simulink model "segway_TP3_sensors"  (R2016a)
settings: Solver=VariableStepAuto  StartTime=t0  StopTime=200  FixedStep=h  RelTol=1e-3
values from neighbouring files (symbols this model uses):
  h = (tf-t0)/N    [init.m]    (also in init_tp3.m)
  l = 10    [init.m]    (also in init_TP1.m = 1; init_TP2_controle.m; init_tp3.m = 5)
undefined symbols (not defined in the file or in its folder): DiscIntNeverNeededParam
libraries: simulink x1
settings Model: Creator=fgaribal  LastModifiedBy=fgaribal

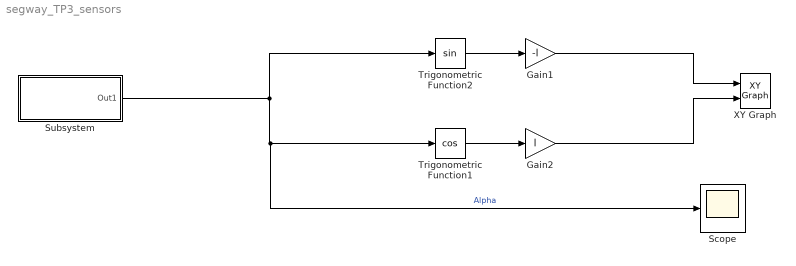
== system segway_TP3_sensors ==
  Gain1 : Gain  Gain=-l
  Gain2 : Gain  Gain=l
  Scope : Scope
  Subsystem : Subsystem
  Trigonometric Function1 : Trigonometry  Operator=cos
  Trigonometric Function2 : Trigonometry
  XY Graph : simulink/Sinks/XY Graph  xmin=-l  xmax=l  ymin=-l  ymax=l  st=-1
  wires:
  Trigonometric Function1/1 -> Gain2/1
  Trigonometric Function2/1 -> Gain1/1
  Gain2/1 -> XY Graph/2
  Gain1/1 -> XY Graph/1
  Subsystem/1(Out1) -> Scope/1, Trigonometric Function1/1, Trigonometric Function2/1  "Alpha"

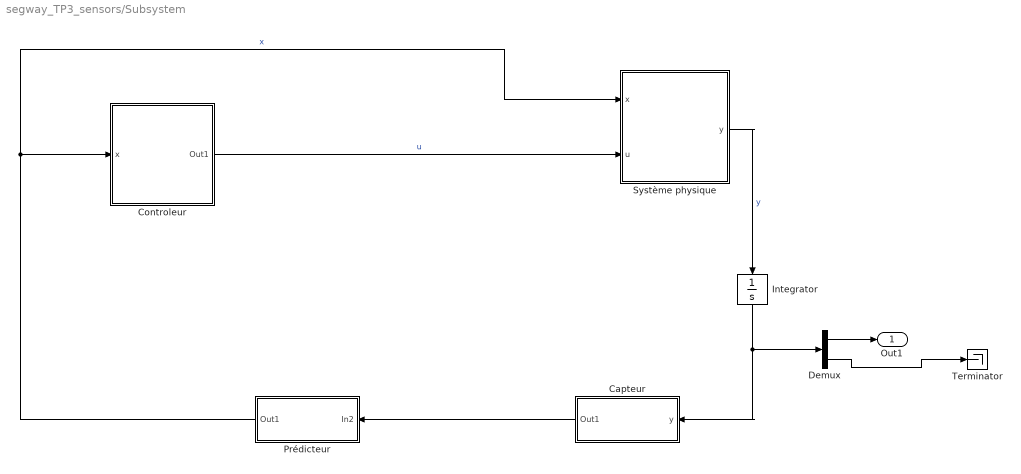
== system segway_TP3_sensors/Subsystem ==
  "Capteur " : Subsystem
  Controleur : Subsystem
  Demux : Demux  Outputs=2
  Integrator : Integrator  InitialCondition=pi/4
  Prédicteur : Subsystem
  Système physique : Subsystem
  Terminator : Terminator
  Out1 : Outport
  wires:
  Controleur/1(Out1) -> Système physique/2(u)  "u"
  Prédicteur/1(Out1) -> Système physique/1(x), Controleur/1(x)  "x"
  Système physique/1(y) -> Integrator/1  "y"
  "Capteur "/1(Out1) -> Prédicteur/1(In2)
  Integrator/1 -> Demux/1, "Capteur "/1(y)
  Demux/1 -> Out1/1
  Demux/2 -> Terminator/1

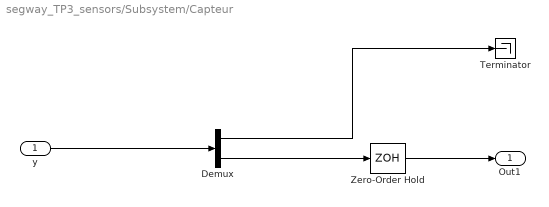
== system segway_TP3_sensors/Subsystem/Capteur  ==
  y : Inport
  Demux : Demux  Outputs=2
  Terminator : Terminator
  Zero-Order Hold : ZeroOrderHold  SampleTime=25*h
  Out1 : Outport
  wires:
  Demux/2 -> Zero-Order Hold/1
  Demux/1 -> Terminator/1
  y/1 -> Demux/1
  Zero-Order Hold/1 -> Out1/1

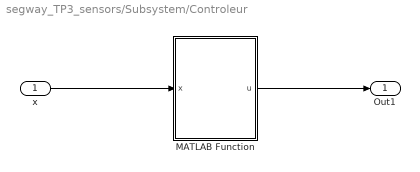
== system segway_TP3_sensors/Subsystem/Controleur ==
  x : Inport
  MATLAB Function : MATLAB Function  TreatAsAtomicUnit=on
  Out1 : Outport
  wires:
  MATLAB Function/1(u) -> Out1/1
  x/1 -> MATLAB Function/1(x)

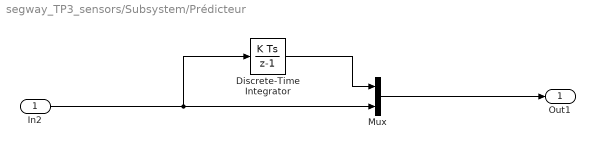
== system segway_TP3_sensors/Subsystem/Prédicteur ==
  In2 : Inport
  Discrete-Time Integrator : DiscreteIntegrator  InitialConditionSetting=State (most efficient)  SampleTime=25*h  ICPrevOutput=DiscIntNeverNeededParam  ICPrevScaledInput=DiscIntNeverNeededParam
  Mux : Mux  Inputs=2
  Out1 : Outport
  wires:
  In2/1 -> Discrete-Time Integrator/1, Mux/2
  Discrete-Time Integrator/1 -> Mux/1
  Mux/1 -> Out1/1

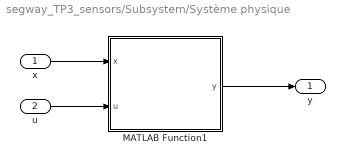
== system segway_TP3_sensors/Subsystem/Système physique ==
  x : Inport
  u : Inport  Port=2
  MATLAB Function1 : MATLAB Function  TreatAsAtomicUnit=on
  y : Outport
  wires:
  MATLAB Function1/1(y) -> y/1
  x/1 -> MATLAB Function1/1(x)
  u/1 -> MATLAB Function1/2(u)

== matlab function segway_TP3_sensors/Subsystem/Système physique/MATLAB Function1 ==
  data: x input; u input; y output
function y = pendule_inverse(x,u)
    g = 9.81;
    l = 10;
    
    y = zeros(2,1);
    y(1) = x(2);
    y(2) = g/l*sin(x(1))-((u*cos(x(1)))/l);
end

== matlab function segway_TP3_sensors/Subsystem/Controleur/MATLAB Function ==
  data: x input; u output
function u = calcul_u(x)
    ue = 0;
    xe = [0;0];
    K = [20;10];
    
    u = ue + K'*(x-xe);
end
